simulink model "Problema2"  (R2016a)
settings: Solver=VariableStepDiscrete  StartTime=0.0  StopTime=200  RelTol=1e-3
undefined symbols (not defined in the file): m, n
settings Model: Creator=Cristina  LastModifiedBy=Cristina

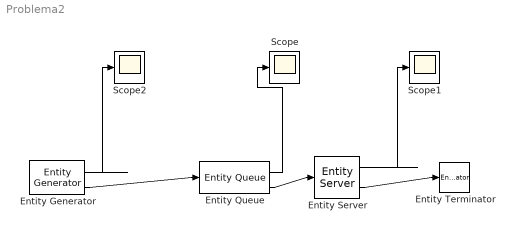
== system Problema2 ==
  Entity Generator : EntityGenerator  OutputPortMessageModes=n,m  IntergenerationTimeAction=dt = 1;  AverageIntergenerationTime=on  EntityType=Structured  EntityTypeName=Entity
      settings: OutputPortMap=o2,o3
  Entity Queue : EntityQueue  InputPortMessageModes=m  OutputPortMessageModes=n,m  NumberEntitiesInBlock=on
      settings: OutputPortMap=o1,o5
  Entity Server : EntityServer  InputPortMessageModes=m  OutputPortMessageModes=n,m  Capacity=1  ServiceTimeSource=MATLAB action  ServiceTimeValue=1.1  ServiceTimeAction=dt = 0.8 + 0.4*rand;  AverageWait=on
      settings: OutputPortMap=o4,o9
  Entity Terminator : EntityTerminator  InputPortMessageModes=m
  Scope : Scope
  Scope1 : Scope
  Scope2 : Scope
  wires:
  Entity Generator/2 -> Entity Queue/1
  Entity Queue/2 -> Entity Server/1
  Entity Server/2 -> Entity Terminator/1
  Entity Queue/1 -> Scope/1
  Entity Server/1 -> Scope1/1
  Entity Generator/1 -> Scope2/1
